simulink model "MathFunction"  (R2020a)
settings: Solver=VariableStepAuto  StartTime=0.0  StopTime=10.0  RelTol=1e-3
undefined symbols (not defined in the file): magnitude
settings Model: Creator=royde  LastModifiedBy=royde

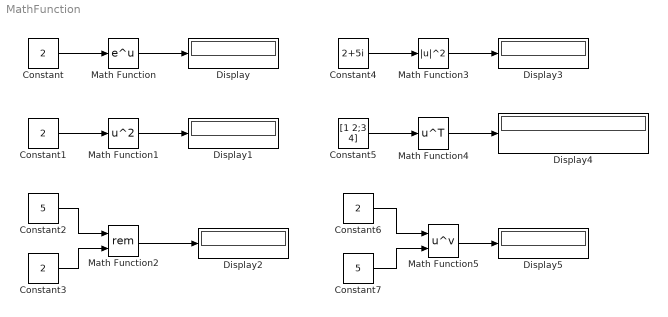
== system MathFunction ==
  Constant{,1,3,6} (4 alike) : Constant  Value=2
  Constant2 : Constant  Value=5
  Constant4 : Constant  Value=2+5i
  Constant5 : Constant  Value=[1 2;3 4]
  Constant7 : Constant  Value=5
  Display{,1..5} (6 alike) : Display
  Math Function : Math  SaturateOnIntegerOverflow=on
  Math Function1 : Math  Operator=square  SaturateOnIntegerOverflow=on
  Math Function2 : Math  Operator=rem  SaturateOnIntegerOverflow=on
  Math Function3 : Math  Operator=magnitude^2  SaturateOnIntegerOverflow=on
  Math Function4 : Math  Operator=transpose  SaturateOnIntegerOverflow=on
  Math Function5 : Math  Operator=pow  SaturateOnIntegerOverflow=on
  wires:
  Constant/1 -> Math Function/1
  Math Function/1 -> Display/1
  Math Function1/1 -> Display1/1
  Constant1/1 -> Math Function1/1
  Constant2/1 -> Math Function2/1
  Math Function2/1 -> Display2/1
  Math Function3/1 -> Display3/1
  Constant4/1 -> Math Function3/1
  Constant3/1 -> Math Function2/2
  Math Function5/1 -> Display5/1
  Constant6/1 -> Math Function5/1
  Constant7/1 -> Math Function5/2
  Constant5/1 -> Math Function4/1
  Math Function4/1 -> Display4/1
